simulink model "reaching_sim"  (R2023b)
settings: Solver=FixedStepAuto  StartTime=0.0  StopTime=inf  FixedStep=time_step  RelTol=1e-3
InitFcn:
  | reaching_init
values from neighbouring files (symbols this model uses):
  coord_home = [0,0]    [reaching_init.m]
  coord_targets = zeros(n_target,2)    [reaching_init.m]
  th = 0.005    [reaching_init.m]
libraries: vrlib x1
settings Model: Creator=davide  LastModifiedBy=Davide

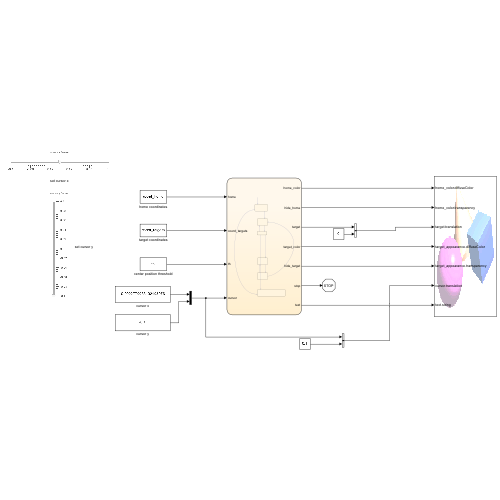
[thumbnail: Simulink's stored preview of the top-level diagram]
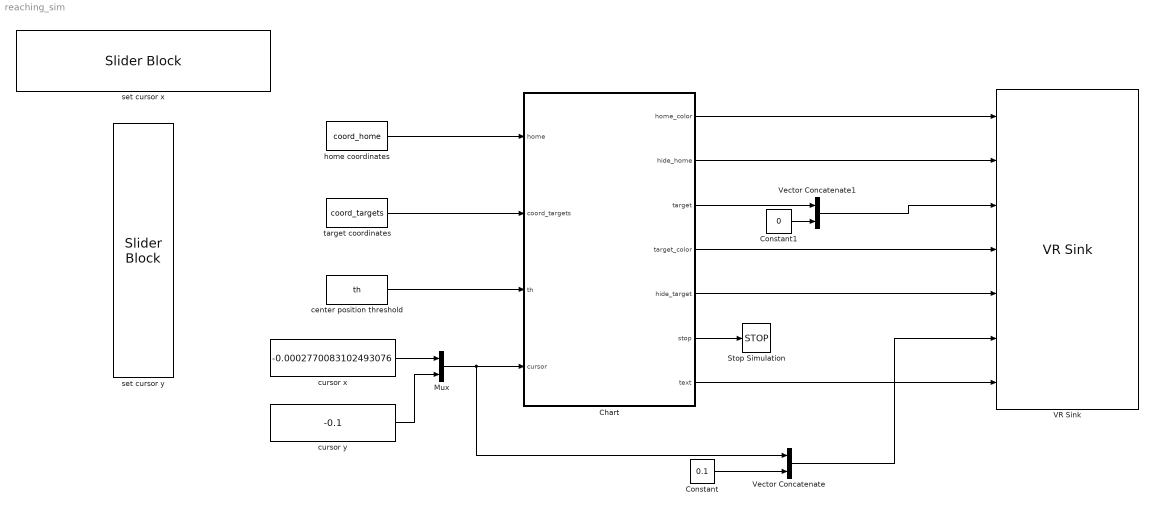
== system reaching_sim ==
  Chart : Stateflow chart  TreatAsAtomicUnit=on
  Constant : Constant  Value=0.1
  Constant1 : Constant  Value=0
  Mux : Mux  Inputs=2
  Stop Simulation : Stop
  VR Sink : vrlib/VR Sink  InstantiateOnLoad=on  SampleTime=0.1  ViewEnable=on  RemoteChange=off  RemoteView=off  FieldsWritten=home_color.diffuseColor.3.1.1.double#home_color.transparency.1.1.1.double#target.translation.3.1.1.double#target_appearance.diffuseColor.3.1.1.double#target_appearance.transparency.1.1.1.double#cursor.translation.3.1.1.double#text.string.1.-1.1.char  WorldFileName=a3_world.wrl  AutoView=off  VideoDimensions=[]  AllowVariableSize=off
  Vector Concatenate : Concatenate
  Vector Concatenate1 : Concatenate
  center position threshold : Constant  Value=th
  cursor x : Constant  Value=-0.0002770083102493076
  cursor y : Constant  Value=-0.1
  home coordinates : Constant  Value=coord_home
  set cursor x : SliderBlock  ScaleMin=-0.1  ScaleMax=0.1
  set cursor y : SliderBlock  ScaleMin=-0.1  ScaleMax=0.1
  target coordinates : Constant  Value=coord_targets
  wires:
  target coordinates/1 -> Chart/2(coord_targets)
  center position threshold/1 -> Chart/3(th)
  home coordinates/1 -> Chart/1(home)
  cursor x/1 -> Mux/1
  cursor y/1 -> Mux/2
  Mux/1 -> Vector Concatenate/1, Chart/4(cursor)
  Constant/1 -> Vector Concatenate/2
  Constant1/1 -> Vector Concatenate1/2
  Chart/3(target) -> Vector Concatenate1/1
  Chart/6(stop) -> Stop Simulation/1
  Chart/2(hide_home) -> VR Sink/2
  Vector Concatenate1/1 -> VR Sink/3
  Chart/4(target_color) -> VR Sink/4
  Chart/5(hide_target) -> VR Sink/5
  Vector Concatenate/1 -> VR Sink/6
  Chart/7(text) -> VR Sink/7
  Chart/1(home_color) -> VR Sink/1

== stateflow chart reaching_sim/Chart ==
  state start
  state goToHome
  state home
  state goToTarget
  state target
  state end
    text = string("Well done!");
    stop = true;
  (default) -> start : {targets = coord_targets;
      |   stop = false;
      |   text = "";}
  start -> end [order 1] : [size(targets,1)==0]
  start -> goToHome [order 2] : {hide_home = false;
      | hide_target = true;
      | home_color = [1,0.6,0];}
  target -> goToHome [order 2] : after(1,sec)
      | {
      |   hide_target = true;
      |   hide_home = false;
      |   home_color = [1,0.6,0];
      | }
  home -> goToHome [order 1] : [norm(cursor-home) >= th]
      | {home_color = [1,0.6,0];}
  goToHome -> home : [norm(cursor-home) < th]
      | {home_color = [0,0.8,0];}
  home -> end [order 3] : [size(targets,1) == 0]
  home -> goToTarget [order 2] : after(2,sec)
      | [size(targets,1)>0]
      | {
      |   target = targets(1,1:2)';
      |   targets(1,:) = [];
      |   target_color = [1,0,0];
      |   hide_home = true;
      |   hide_target = false;
      | }
  target -> goToTarget [order 1] : [norm(cursor-target) >= th]
      | {target_color=[1,0,0];}
  goToTarget -> target : [norm(cursor-target) < th]
      | {
      |   target_color=[0,1,0];
      | }
  data: home_color output; home input; targets local double size=[8,2]; coord_targets input; th input double; cursor input; hide_home output; target output double size=[2,1]; target_color output; hide_target output; stop output; text output string
